simulink model "conttest_discrete_PID"  (Simulink 6.5)
settings: Solver=FixedStepDiscrete  StartTime=0.0  StopTime=max(T)  FixedStep=delta_t  RelTol=1e-3
values from neighbouring files (symbols this model uses):
  AK = PID.A    [PIDforsim.m]
  BK = PID.B    [PIDforsim.m]
  CK = PID.C    [PIDforsim.m]
  delta_t = 1e-4    (= 0.0001)    [makesim.m]    (also in runsim_PID.m)
  DK = PID.D    [PIDforsim.m]
  Gd = c2d(G,delta_t,'tustin')    [makesim.m]
  PSlimits = PSlimits(1:size(K,1))    [makesim.m]
settings Model: Creator=asharma  LastModifiedBy=asharma  ExtModeTrigMode=oneshot  ExtModeArmWhenConnect=off  ExtModeAutoUpdateStatusClock=off
settings DataIOCC: LimitDataPoints=off
settings OptimizationCC: BlockReduction=off  BooleanDataType=off
settings DebuggingCC: SolverPrmCheckMsg=none  MultiTaskDSMMsg=warning  MultiTaskCondExecSysMsg=none  StrictBusMsg=None
settings HardwareCC: TargetUnknown=on
settings RTWCC: IncludeERTFirstTime=on

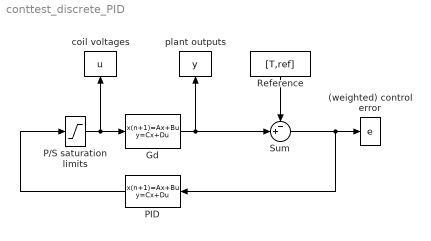
== system conttest_discrete_PID ==
  (weighted) control error : ToWorkspace  VariableName=e  SampleTime=-1  SaveFormat=Array
  Gd : DiscreteStateSpace  A=Gd.A  B=Gd.B  C=Gd.C  D=Gd.D  SampleTime=delta_t
  P/S saturation limits : Saturate  UpperLimit=PSlimits  LowerLimit=-PSlimits
  PID : DiscreteStateSpace  Orientation=left  A=AK  B=BK  C=CK  D=DK  SampleTime=1e-4
  Reference : FromWorkspace  Orientation=down  VariableName=[T,ref]  Interpolate=off  OutputAfterFinalValue=Setting to zero
  Sum : Sum  Inputs=-+|  SaturateOnIntegerOverflow=on  InputSameDT=on
  coil voltages : ToWorkspace  VariableName=u  SampleTime=-1  SaveFormat=Array
      settings: Orientation=up
  plant outputs : ToWorkspace  VariableName=y  SampleTime=-1  SaveFormat=Array
      settings: Orientation=up
  wires:
  Reference/1 -> Sum/1
  Gd/1 -> Sum/2, plant outputs/1
  P/S saturation limits/1 -> Gd/1, coil voltages/1
  PID/1 -> P/S saturation limits/1
  Sum/1 -> (weighted) control error/1, PID/1
